simulink model "roll_sim"  (R2021b)
settings: Solver=VariableStepAuto  StartTime=0.0  StopTime=20  RelTol=1e-3
values from neighbouring files (symbols this model uses):
  J_ph = 0.04969    [lab3_workspace.m]
  K_f = 0.0784    [lab3_workspace.m]
  K_ph_d = ((J_ph*(2*z_r*wn_r))/(K_f*l_h))*0.5    [lab3_workspace.m]
  K_ph_p = (J_ph*wn_r^2)/(K_f*l_h)    [lab3_workspace.m]
  l_h = 0.18    [lab3_workspace.m]
settings Model: Creator=DSDLn  LastModifiedBy=DSDLn

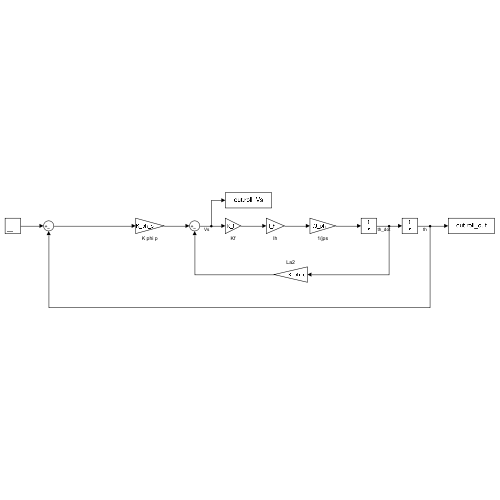
[thumbnail: Simulink's stored preview of the top-level diagram]
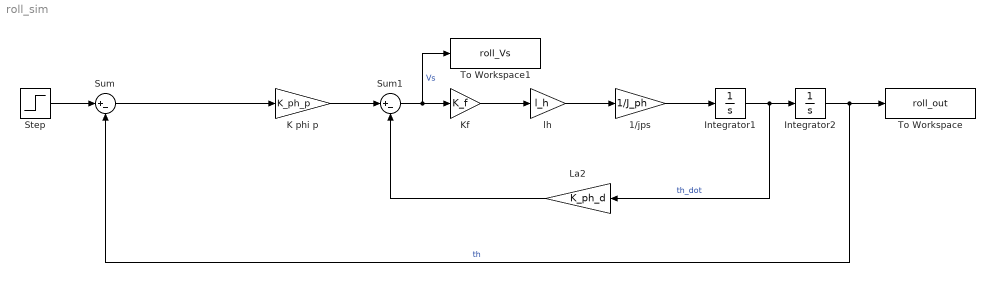
== system roll_sim ==
  1/jps : Gain  Gain=1/J_ph
  Integrator1 : Integrator
  Integrator2 : Integrator
  K phi p : Gain  Gain=K_ph_p
  Kf : Gain  Gain=K_f
  La2 : Gain  Gain=K_ph_d
  Step : Step  Time=0  After=deg2rad(10)  SampleTime=0.01
  Sum : Sum  Inputs=|+-
  Sum1 : Sum  Inputs=|+-
  To Workspace : ToWorkspace  VariableName=roll_out  SampleTime=-1
  To Workspace1 : ToWorkspace  VariableName=roll_Vs  SampleTime=-1
  lh : Gain  Gain=l_h
  wires:
  Step/1 -> Sum/1
  Sum1/1 -> To Workspace1/1, Kf/1  "Vs"
  Kf/1 -> lh/1
  1/jps/1 -> Integrator1/1
  lh/1 -> 1/jps/1
  Integrator1/1 -> Integrator2/1, La2/1  "th_dot"
  Integrator2/1 -> To Workspace/1, Sum/2  "th"
  Sum/1 -> K phi p/1
  La2/1 -> Sum1/2
  K phi p/1 -> Sum1/1
